simulink model "MagLev"  (R2018b)
settings: Solver=FixedStepAuto  StartTime=0.0  StopTime=inf  RelTol=1e-3  EnableMultiTasking=on
undefined symbols (not defined in the file): magnitude, Standard_Devices, UDP_Protocol
libraries: sldrtlib x2, fod x1
settings Model: SimulationMode=external  Creator=Alex  LastModifiedBy=Aleksei Tepljakov
settings DataIOCC: LimitDataPoints=on  SaveFormat=Array
settings OptimizationCC: ExpressionDepthLimit=2147483647
settings DebuggingCC: AlgebraicLoopMsg=error  UnderspecifiedInitializationDetection=Classic  MergeDetectMultiDrivingBlocksExec=none  SolverPrmCheckMsg=warning  StateNameClashWarn=warning  SFUnexpectedBacktrackingDiag=warning  SFNoUnconditionalDefaultTransitionDiag=warning  SFExecutionAtInitializationDiag=none
settings ModelReferenceCC: PropagateSignalLabelsOutOfModel=off
settings SFSimCC: SimUseLocalCustomCode=off
settings RTWCC: SystemTargetFile=sldrt.tlc  TemplateMakefile=sldrt.tmf  Description=Simulink Desktop Real-Time  RTWUseLocalCustomCode=off  RTWCompilerOptimization=on
settings CodeAppCC: MaxIdLength=95  StateflowObjectComments=on
settings SimulinkDesktopRealTimeCC: TargetPreCompLibLocation=C:\Program Files\MATLAB\R2018b\toolbox\sldrt\lib\win64  TargetLangStandard=C89/C90 (ANSI)  SupportVariableSizeSignals=off  PreserveStateflowLocalDataDimensions=off
settings ConfigComp: CovMetricSettings=dw  CovHtmlReporting=on  CovSaveCumulativeToWorkspaceVar=on  CovSaveSingleToWorkspaceVar=on  CovExternalEMLEnable=off  CovSFcnEnable=off

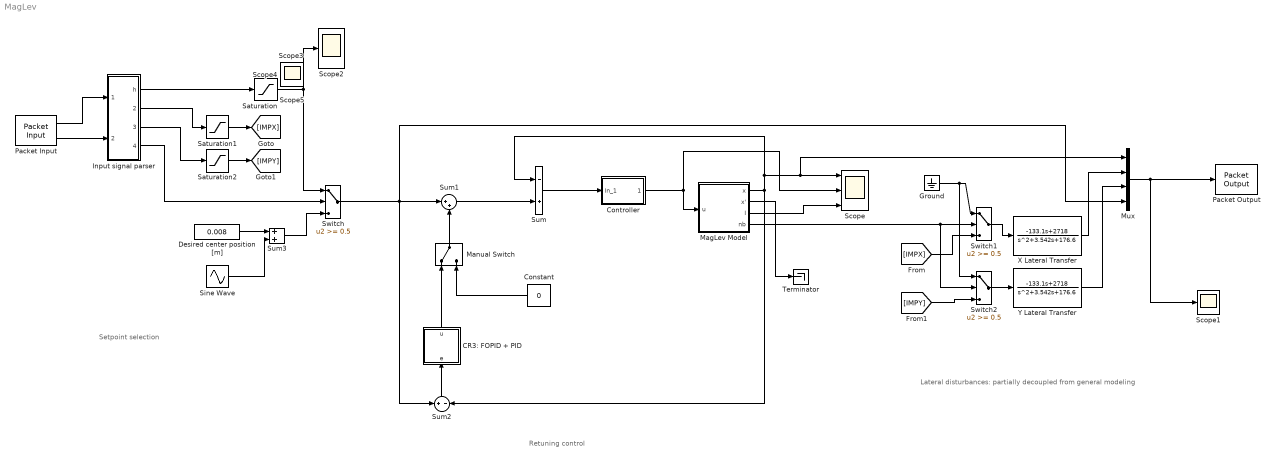
== system MagLev ==
  note: Lateral disturbances: partially
      | decoupled from general modeling
  note: Retuning control
  note: Setpoint selection
  CR3: FOPID + PID : Subsystem  mask{Kps=-54.444, Kis=-47.6078, lambda=0.82, Kds=-3.7773, mu=0.98, Kp=-39, Ki=-10, Kd=-2.05, Ts=0.001}
      mask prompts: Kps "Kp*"; Kis "Ki*"; Kds "Kd*"; Ts "Sampling interval"
  Constant : Constant  Value=0
  Controller : Subsystem  mask(PID(2) Controller){P=-39, I=-10, D=-2.05, T0=0.001}
      mask prompts: P "Proportional:"; I "Integral:"; D "Derivative:"; T0 "Sample Time:"
      mask help:
      | Enter Proportional(P), Integral(I), and Derivative(D) and divisor (N) terms.
      | P+I/s+Ds/(1/Ns+1)
      mask Help: This block implements a PID controller where parameters are entered for the Proportional, Integral and Derivative and divisor terms. Unmask this block to see how it works. The derivative term is implemented using an s/(s/N +1)  transfer function block. Making N large can create a "stiff" system.
      mask Display: disp('PID')
  Desired center position [m] : Constant  Value=0.008
  Ground : Ground
  Input signal parser : Subsystem
  MagLev Model : Subsystem  mask{x0=0.0153, m=58.5e-3, u_poly=[-0.3 2.6 -0.047], u_dz=0.0182, c_poly=[0.5756 0.16214 -0.22428 0.0062399 2.8328e-5], nba=0.001}
      mask prompts: x0 "Initial position : x0"; m "Mass of ball : m"; u_poly "Control conversion polynomial"; u_dz "Control dead zone : u_dz"; c_poly "Current/position factor c polynomial"; nba "Near bounds (nb) detection accuracy [m]"
  Manual Switch : ManualSwitch
  Mux : Mux
  Packet Input : sldrtlib/Packet Input  SampleTime=0.001  MaxMissedTicks=10  ShowMissedTicks=off  YieldWhenWaiting=off  DrvName=Standard_Devices/UDP_Protocol  DrvAddress=9977  DrvOptions=[0 9955 49 50 55 46 48 46 48 46 49 0 0 0 0 0 0 0 0 0 0 0 0 0 0 0 0 0 0 0 0 0 0 0 0 0 0 0 0 0 0 0 0 0 0 0 0 0 0 0 0 0 0 0 0 0 0 0 0 0 0 0 0 0 0 0 0 0 0 0 0 0 0 0 0 0 0 0 0 0 0 0 0 0 0 0 0 0 0 0 0 0 0 0 0 0 0 0 0 0 0 0 0 0 0 0 0 0 0 0 0 0 0 0 0 0 0 0 0 0 0 0 0 0 0 0 0 0 0 0 0 0 0 0 0 0 0 0 0 0 0 0 0 0 0 0 0 0 0 0 0 0 0 0 0 0 0 0 0 0 0 0 0 0 0 0 0 0 0 0 0 0 0 0 0 0 0 0 0 0 0 0 0 0 0 0 0 0 0 0 0 0 0 0 0 0 0 0 0 0 0 0 0 0 0 0 0 0 0 0 0 0 0 0 0 0 0 0 0 0 0 0 0 0 0 0 0 0 0 0 0 0 0 0 0 0 0 0 0 0 0 0 0 0 0 0 0 0 0 0 0 0 0 0 0 0]  PacketSize=20*4+3  DataTypes={'20*single', '3*uint8'}  ShowReady=off  ShowError=off  PacketID=1  ByteOrder=1  ShowTimestamp=off
      settings: AttributesFormatString=UDP Protocol [9977]  SourceProductName=Simulink Desktop Real-Time
  Packet Output : sldrtlib/Packet Output  SampleTime=0.001  MaxMissedTicks=10  ShowMissedTicks=off  YieldWhenWaiting=off  DrvName=Standard_Devices/UDP_Protocol  DrvAddress=9999  DrvOptions=[0 9988 49 50 55 46 48 46 48 46 49 0 0 0 0 0 0 0 0 0 0 0 0 0 0 0 0 0 0 0 0 0 0 0 0 0 0 0 0 0 0 0 0 0 0 0 0 0 0 0 0 0 0 0 0 0 0 0 0 0 0 0 0 0 0 0 0 0 0 0 0 0 0 0 0 0 0 0 0 0 0 0 0 0 0 0 0 0 0 0 0 0 0 0 0 0 0 0 0 0 0 0 0 0 0 0 0 0 0 0 0 0 0 0 0 0 0 0 0 0 0 0 0 0 0 0 0 0 0 0 0 0 0 0 0 0 0 0 0 0 0 0 0 0 0 0 0 0 0 0 0 0 0 0 0 0 0 0 0 0 0 0 0 0 0 0 0 0 0 0 0 0 0 0 0 0 0 0 0 0 0 0 0 0 0 0 0 0 0 0 0 0 0 0 0 0 0 0 0 0 0 0 0 0 0 0 0 0 0 0 0 0 0 0 0 0 0 0 0 0 0 0 0 0 0 0 0 0 0 0 0 0 0 0 0 0 0 0 0 0 0 0 0 0 0 0 0 0 0 0 0 0 0 0 0 0]  PacketSize=4*4  DataTypes='4*single'  ShowReady=off  ShowError=off  PacketID=1  ByteOrder=1  InitialValue=[]  FinalValue=[]
      settings: AttributesFormatString=UDP Protocol [9999]  SourceProductName=Simulink Desktop Real-Time
  Saturation : Saturate  UpperLimit=0.012  LowerLimit=0.007
  Saturation1 : Saturate  UpperLimit=1e-1  LowerLimit=-1e-1
  Saturation2 : Saturate  UpperLimit=1e-1  LowerLimit=-1e-1
  Scope : Scope  NumInputPorts=3
  Scope{1..5} (5 alike) : Scope
  Sine Wave : Sin  Amplitude=0.0015  Frequency=2  SampleTime=0
  Sum : Sum  Inputs=-+  SaturateOnIntegerOverflow=on  InputSameDT=on  OutDataTypeStr=Inherit: Same as first input
  Sum1 : Sum  Inputs=|++  SaturateOnIntegerOverflow=on  InputSameDT=on  OutDataTypeStr=Inherit: Same as first input
  Sum2 : Sum  Inputs=+|-  SaturateOnIntegerOverflow=on  InputSameDT=on  OutDataTypeStr=Inherit: Same as first input
  Sum3 : Sum  SaturateOnIntegerOverflow=on  InputSameDT=on  OutDataTypeStr=Inherit: Same as first input
  Switch : Switch  Threshold=0.5  SaturateOnIntegerOverflow=on  InputSameDT=on
  Switch1 : Switch  Threshold=0.5  SaturateOnIntegerOverflow=on  InputSameDT=on
  Switch2 : Switch  Threshold=0.5  SaturateOnIntegerOverflow=on  InputSameDT=on
  Terminator : Terminator
  "X Lateral Transfer " : TransferFcn  Numerator=[-133.1 2718]  Denominator=[1 3.542 176.6]
  Y Lateral Transfer : TransferFcn  Numerator=[-133.1 2718]  Denominator=[1 3.542 176.6]
  wires:
  Controller/1(Out_1) -> MagLev Model/1(u), Scope/2
  MagLev Model/3(I) -> Scope/3
  Sum/1 -> Controller/1(In_1)
  Switch/1 -> Mux/4, Sum2/1, Sum1/1
  CR3: FOPID + PID/1(u) -> Manual Switch/1
  Sum1/1 -> Sum/2
  Sum2/1 -> CR3: FOPID + PID/1(e)
  Constant/1 -> Manual Switch/2
  Manual Switch/1 -> Sum1/2
  MagLev Model/1(x) -> Sum/1, Mux/1, Scope/1, Sum2/2
  MagLev Model/2(x') -> Terminator/1
  Desired center position [m]/1 -> Sum3/1
  Sine Wave/1 -> Sum3/2
  Mux/1 -> Scope1/1, Packet Output/1
  "X Lateral Transfer "/1 -> Mux/2
  Y Lateral Transfer/1 -> Mux/3
  Packet Input/1 -> Input signal parser/1(In1)
  Packet Input/2 -> Input signal parser/2(In2)
  Input signal parser/2(impX) -> Saturation1/1
  Input signal parser/3(impY) -> Saturation2/1
  [IMPY] -> Switch2/3
  [IMPX] -> Switch1/3
  Input signal parser/1(h) -> Saturation/1
  Input signal parser/4(mode) -> Switch/2
  Sum3/1 -> Switch/3
  Switch1/1 -> "X Lateral Transfer "/1
  Switch2/1 -> Y Lateral Transfer/1
  MagLev Model/4(nb) -> Switch2/2, Switch1/2
  Ground/1 -> Switch2/1, Switch1/1
  Saturation/1 -> Switch/1, Scope2/1
  Saturation1/1 -> [IMPX]
  Saturation2/1 -> [IMPY]

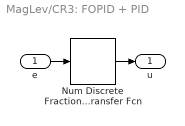
== system MagLev/CR3: FOPID + PID ==
  e : Inport
  Num Discrete Fractional Transfer Fcn : fod/Num Discrete Fractional Transfer Fcn  b=[Kds Kis -Kd (Kps-Kp) -Ki]  nb=[mu+1 1-lambda 2 1 0]  a=[Kd Kp Ki]  na=[2 1 0]  freqRange=[0.001, 1000]  approxNum=5  useRef=off  dscrMethod=Matched  wc=0  ts=Ts
      settings: SourceProductName=FOMCON Toolbox
  u : Outport
  wires:
  e/1 -> Num Discrete Fractional Transfer Fcn/1
  Num Discrete Fractional Transfer Fcn/1 -> u/1

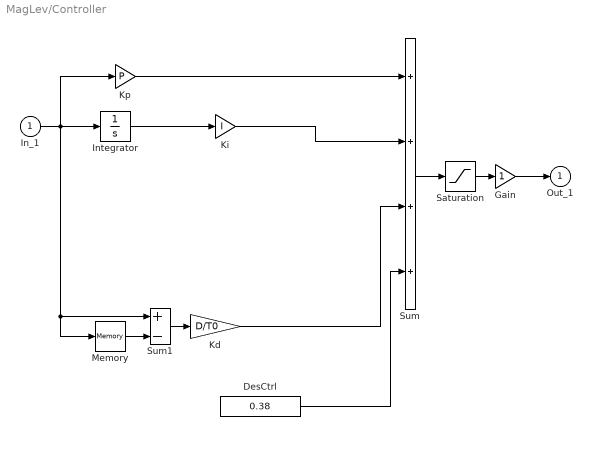
== system MagLev/Controller ==
  In_1 : Inport
  DesCtrl : Constant  Value=0.38
  Gain : Gain  SaturateOnIntegerOverflow=on  OutDataTypeStr=Inherit: Same as input  ParamDataTypeStr=Inherit: Same as input
  Integrator : Integrator  InitialCondition=0*4e-5  LimitOutput=on  UpperSaturationLimit=1  LowerSaturationLimit=-1
  Kd : Gain  Gain=D/T0  SaturateOnIntegerOverflow=on  OutDataTypeStr=Inherit: Same as input  ParamDataTypeStr=Inherit: Same as input
  Ki : Gain  Gain=I  SaturateOnIntegerOverflow=on  OutDataTypeStr=Inherit: Same as input  ParamDataTypeStr=Inherit: Same as input
  Kp : Gain  Gain=P  SaturateOnIntegerOverflow=on  OutDataTypeStr=Inherit: Same as input  ParamDataTypeStr=Inherit: Same as input
  Memory : Memory
  Saturation : Saturate  UpperLimit=1  LowerLimit=0
  Sum : Sum  Inputs=++++  SaturateOnIntegerOverflow=on  InputSameDT=on  OutDataTypeStr=Inherit: Same as first input
  Sum1 : Sum  Inputs=+-  SaturateOnIntegerOverflow=on  InputSameDT=on  OutDataTypeStr=Inherit: Same as first input
  Out_1 : Outport  InitialOutput=0
  wires:
  Ki/1 -> Sum/2
  Integrator/1 -> Ki/1
  Sum/1 -> Saturation/1
  In_1/1 -> Kp/1, Memory/1, Sum1/1, Integrator/1
  Memory/1 -> Sum1/2
  Sum1/1 -> Kd/1
  DesCtrl/1 -> Sum/4
  Saturation/1 -> Gain/1
  Kp/1 -> Sum/1
  Kd/1 -> Sum/3
  Gain/1 -> Out_1/1

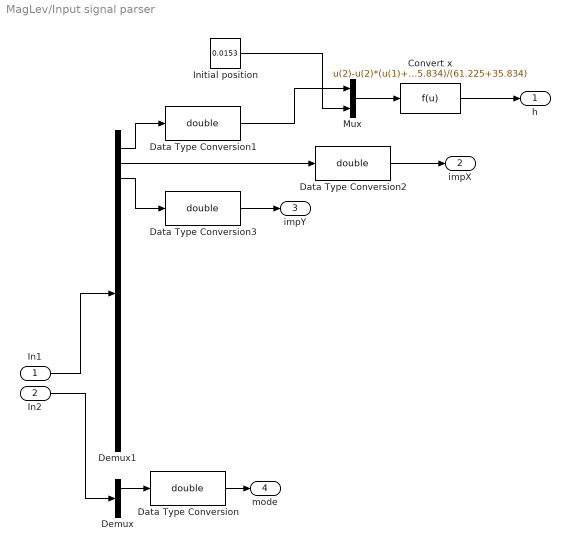
== system MagLev/Input signal parser ==
  In1 : Inport
  In2 : Inport  Port=2
  "Convert x " : Fcn  Expr=u(2)-u(2)*(u(1)+35.834)/(61.225+35.834)
  Data Type Conversion{,1..3} (4 alike) : DataTypeConversion  OutDataTypeStr=double
  Demux : Demux  Outputs=3
  Demux1 : Demux  Outputs=20
  "Initial position " : Constant  Value=0.0153
  Mux : Mux  Inputs=2
  h : Outport
  impX : Outport  Port=2
  impY : Outport  Port=3
  mode : Outport  Port=4
  wires:
  Demux/1 -> Data Type Conversion/1
  Demux1/2 -> Data Type Conversion2/1
  Demux1/1 -> Data Type Conversion1/1
  Demux1/3 -> Data Type Conversion3/1
  In2/1 -> Demux/1
  In1/1 -> Demux1/1
  Data Type Conversion/1 -> mode/1
  Data Type Conversion2/1 -> impX/1
  Data Type Conversion3/1 -> impY/1
  "Convert x "/1 -> h/1
  "Initial position "/1 -> Mux/2
  Data Type Conversion1/1 -> Mux/1
  Mux/1 -> "Convert x "/1

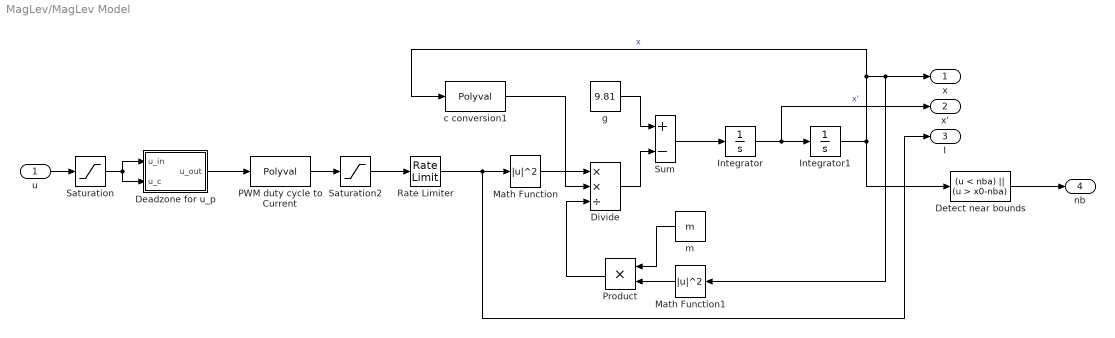
== system MagLev/MagLev Model ==
  u : Inport
  Deadzone for u_p : Subsystem  mask{ud_high=u_dz}
      mask prompts: ud_high "Deadzone range upper limit in [0; ud_high]"
  Detect near bounds : Fcn  Expr=(u < nba) || (u > x0-nba)
  Divide : Product  Inputs=**/
  Integrator : Integrator  UpperSaturationLimit=1  LowerSaturationLimit=-1
  Integrator1 : Integrator  InitialCondition=x0  LimitOutput=on  UpperSaturationLimit=x0  LowerSaturationLimit=1e-5
  Math Function : Math  Operator=magnitude^2  SaturateOnIntegerOverflow=on
  Math Function1 : Math  Operator=magnitude^2  SaturateOnIntegerOverflow=on
  PWM duty cycle to Current : Polyval  Coefs=u_poly
  Product : Product  RndMeth=Zero
  Rate Limiter : RateLimiter  RisingSlewLimit=56.4  FallingSlewLimit=-56.4  SampleTimeMode=inherited
  Saturation : Saturate  UpperLimit=1  LowerLimit=0
  Saturation2 : Saturate  UpperLimit=Inf  LowerLimit=0
  Sum : Sum  Inputs=+-
  c conversion1 : Polyval  Coefs=c_poly
  g : Constant  Value=9.81
  m : Constant  Value=m
  x : Outport
  x' : Outport  Port=2
  I : Outport  Port=3
  nb : Outport  Port=4
  wires:
  Deadzone for u_p/1(u_out) -> PWM duty cycle to Current/1
  Saturation/1 -> Deadzone for u_p/2(u_c), Deadzone for u_p/1(u_in)
  Integrator/1 -> Integrator1/1, x'/1  "x'"
  Divide/1 -> Sum/2
  Integrator1/1 -> Detect near bounds/1, c conversion1/1, x/1, Math Function1/1  "x"
  g/1 -> Sum/1
  u/1 -> Saturation/1
  Math Function/1 -> Divide/1
  PWM duty cycle to Current/1 -> Saturation2/1
  Product/1 -> Divide/3
  Math Function1/1 -> Product/2
  m/1 -> Product/1
  Sum/1 -> Integrator/1
  c conversion1/1 -> Divide/2
  Saturation2/1 -> Rate Limiter/1
  Rate Limiter/1 -> Math Function/1, I/1
  Detect near bounds/1 -> nb/1

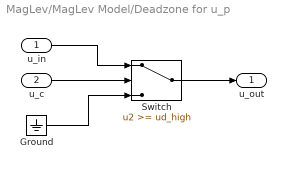
== system MagLev/MagLev Model/Deadzone for u_p ==
  u_in : Inport
  u_c : Inport  Port=2
  Ground : Ground
  Switch : Switch  Threshold=ud_high
  u_out : Outport
  wires:
  u_in/1 -> Switch/1
  Switch/1 -> u_out/1
  Ground/1 -> Switch/3
  u_c/1 -> Switch/2
